simulink library "thc"  (R2021b)
settings: Solver=VariableStepAuto  StartTime=0.0  StopTime=10.0  RelTol=1e-3
undefined symbols (not defined in the file or in its folder): ATHC_APTCQA_X_C, ATHC_APTCQB_X_C, ATHC_dAy_X_C, ATHC_Qeq_X_kmh, ATHC_VbaseC_X_C, ATHC_VbaseC_Y_W, ATHC_VbaseD_X_C, ATHC_VbaseH_X_C, FALSE, KTHC_ACMaxMinT_sec, KTHC_aDeice_K, KTHC_AGSDefLv_K, KTHC_AGSLv1_K, KTHC_AGSLv2_K, KTHC_AGSLv3_K, KTHC_AGSLv4_K, KTHC_AGSLv5_K, KTHC_AirIntUpdateT_sec, KTHC_APTCOneZoneMax_W, KTHC_APTCPeriod_cnt, KTHC_APTCPWMEN_flg, KTHC_APTCQMaxC_W, KTHC_APTCQminC_W, KTHC_APTCQminD_W, KTHC_APTCQminRe1_W, KTHC_APTCQminRe_W, KTHC_APTCQoffT_cnt, KTHC_APTCQonT_cnt, KTHC_APTCRiLeMaxDff_W, KTHC_APTCRiLeMinDff_W, KTHC_BatInTempDef_C, KTHC_bDeice_K, KTHC_CompMaxDeice_rpm, KTHC_CompMinDeice_rpm, KTHC_CompSotxvOp_K, KTHC_CompSotxvOpLow_rpm, KTHC_CompSpdmax_rpm, KTHC_CompSpdmaxBC1_rpm, KTHC_CompSpdmaxBC_rpm, KTHC_CompSpdmid1_rpm, KTHC_CompSpdmid2_rpm, KTHC_CompSpdmid3_rpm, KTHC_CompSpdmid_rpm, KTHC_CompSpdmin_rpm, KTHC_DAPTCQ1_W, KTHC_DAPTCQ2_W, KTHC_DAPTCQ3_W, KTHC_DcChSetTemp_C, KTHC_DehumidityEN_flg, KTHC_DeiceCycTime_K, KTHC_DriveLevelWPTCBAH1_W, KTHC_DriveLevelWPTCBAH2_W, KTHC_DriveLevelWPTCBAH3_W, KTHC_DriveLevelWPTCBAH4_W, KTHC_DriveT1MinBAH_C, KTHC_DriveT2MaxBAH_C, KTHC_DriveT2MinBAH_C, KTHC_DriveT3MaxBAH_C, KTHC_DriveT3MinBAH_C, KTHC_DriveT4MaxBAH_C ... (+372)
libraries: simulink x140
(part 8 of 10)

== stateflow chart thc/THC/ThermalControl/THCM_Conctrl/BlowerCtrl/Enabled Subsystem1/Chart2 ==
  state Voffset [parallel]
    settings: executionOrder=2
    state ACOFF
      state POWERon
        en:Voffset=Vmanual;
        du:Voffset=Vmanual;
      state OFF
        en:Voffset=0;
      (default) -> (junction 8)
      (junction 8) -> POWERon [order 2]
      (junction 8) -> OFF [order 1] : [CabinMode==0||....
          | PwrSta<=3]
      OFF -> POWERon : [CabinMode~=0&&PwrSta>3]
      POWERon -> OFF : [CabinMode==0||....
          | PwrSta<=3]
    state ACON
      state Defrst
        state Manual
          en:Voffset=Vmanual;
          du:Voffset=Vmanual;
        state Auto
          en:Voffset=KTHC_VBlowerdfog_K;
        (default) -> (junction 56)
        (junction 56) -> Voffset.ACON.Defrst.Auto [order 1] : [ACAuto]
        (junction 56) -> Voffset.ACON.Defrst.Manual [order 2]
        Voffset.ACON.Defrst.Manual -> Voffset.ACON.Defrst.Auto : [ACAuto]
        Voffset.ACON.Defrst.Auto -> Voffset.ACON.Defrst.Manual : [!ACAuto]
      state DefrstOFF
        state Auto
          state DontCorrect3
            en:Voffset=KTHC_VBlowerSetLow_K;
          state Vbase1
            en:Voffset=KTHC_VBlowerDcCh_K;
          state Vbase
            en:Voffset=Vbase;
            du:Voffset=Vbase;
          (default) -> (junction 105)
          (junction 105) -> DontCorrect3 [order 1] : [CabinMode==3&&....
              | (ACSubMode==6||ACSubMode==7||ACSubMode==0)]
          Voffset.ACON.DefrstOFF.Auto -> (junction 105) [order 1] : [hasChanged(CabinMode)||....
              | hasChanged(ACSubMode)]
          (junction 105) -> (junction 304) [order 2]
          (junction 304) -> Vbase1 [order 1] : [CabinMode==11]
          (junction 304) -> (junction 293) [order 2]
          (junction 293) -> Voffset.ACON.DefrstOFF.Auto.Vbase
        state Manual
          state DontCorrect
            en:Voffset=Vmanual;
            du:Voffset=Vmanual;
          state Vbase
            en:Voffset=Vbase;
            du:Voffset=Vbase;
          (default) -> (junction 83)
          Voffset.ACON.DefrstOFF.Manual -> (junction 83) [order 1] : [hasChanged(CabinMode)||....
              | hasChanged(ACSubMode)]
          (junction 83) -> DontCorrect [order 1] : [(CabinMode==3&&ACSubMode>=4)||CabinMode==7]
          (junction 83) -> (junction 91) [order 2]
          (junction 91) -> Voffset.ACON.DefrstOFF.Manual.Vbase
        (default) -> (junction 76)
        (junction 76) -> Voffset.ACON.DefrstOFF.Manual [order 2]
        (junction 76) -> Voffset.ACON.DefrstOFF.Auto [order 1] : [ACAuto]
        Voffset.ACON.DefrstOFF.Manual -> Voffset.ACON.DefrstOFF.Auto [order 1] : [ACAuto]
        Voffset.ACON.DefrstOFF.Auto -> Voffset.ACON.DefrstOFF.Manual [order 1] : [!ACAuto]
      (default) -> (junction 58)
      (junction 58) -> Defrst [order 1] : [DfrstReq]
      (junction 58) -> DefrstOFF [order 2]
      DefrstOFF -> Defrst : [DfrstReq]
      Defrst -> DefrstOFF : [!DfrstReq]
    (default) -> ACOFF
    ACOFF -> ACON : [CabinMode>2&&....
        | (CabinMode!=10||....
        | ACSubMode!=1)]
    ACON -> ACOFF : [CabinMode<=2||....
        | (CabinMode==10&&....
        | ACSubMode==1)]
  state VBase [parallel]
    settings: executionOrder=1
    state Cooling
      en:Vbase=VbaseC;
      du:Vbase=VbaseC;
    state Dehumidity
      en:Vbase=VbaseD;
      du:Vbase=VbaseD;
    state Heating
      en:Vbase=VbaseH;
      du:Vbase=VbaseH;
    state Vmanual
      en:Vbase=Vmanual;
      du:Vbase=Vmanual;
    (default) -> (junction 250)
    (junction 254) -> Cooling [order 1] : [CabinMode==3||....
        | (CabinMode==6&&ACSubMode==2)]
    VBase -> (junction 250) : [hasChanged(CabinMode)||....
        | hasChanged(ACAuto)]
    (junction 250) -> (junction 254) [order 1] : [ACAuto]
    (junction 250) -> Vmanual [order 2]
    (junction 254) -> (junction 258) [order 2]
    (junction 258) -> Dehumidity [order 1] : [CabinMode>3&&CabinMode<8]
    (junction 258) -> (junction 263) [order 2]
    (junction 263) -> Heating [order 1] : [CabinMode>=8]
    (junction 263) -> Vmanual [order 2]
  data: ACAuto input; ACSubMode input; CabinMode input; DfrstReq input; VbaseC input; VbaseD input; VbaseH input; Vmanual input; Vbase local double; Voffset output; PwrSta input; KTHC_VBlowerdfog_K input; KTHC_VBlowerMin_K input; KTHC_VBlowerMid_K input; KTHC_VBlowerDcCh_K input; KTHC_VBlowerSetLow_K input

== stateflow chart thc/THC/ThermalControl/THCM_Conctrl/CompCtrl/Enabled Subsystem/Chart ==
  state LV1
    en:DTymin=KTHC_DTymin1_K;
  state LV2
    en:DTymin=KTHC_DTymin2_K;
  state LV3
    en:DTymin=KTHC_DTymin3_K;
  state LV4
    en:DTymin=KTHC_DTymin4_K;
  state LV5
    en:DTymin=KTHC_DTymin5_K;
  (default) -> (junction 8)
  (junction 8) -> LV1 [order 1] : [Tamb<KTHC_T1Maxamb_C]
  (junction 8) -> (junction 9) [order 2]
  LV1 -> LV2 : [Tamb>KTHC_T1Maxamb_C]
  LV2 -> LV1 [order 2] : [Tamb<KTHC_T2Minamb_C]
  (junction 9) -> LV2 [order 1] : [Tamb<KTHC_T2Maxamb_C]
  (junction 9) -> (junction 10) [order 2]
  LV2 -> LV3 [order 1] : [Tamb>KTHC_T2Maxamb_C]
  LV3 -> LV2 [order 2] : [Tamb<KTHC_T3Minamb_C]
  (junction 10) -> LV3 [order 1] : [Tamb<KTHC_T3Maxamb_C]
  (junction 10) -> (junction 11) [order 2]
  LV3 -> LV4 [order 1] : [Tamb>KTHC_T3Maxamb_C]
  LV4 -> LV3 [order 2] : [Tamb<KTHC_T4Minamb_C]
  (junction 11) -> LV4 [order 1] : [Tamb<KTHC_T4Maxamb_C]
  (junction 11) -> (junction 12) [order 2]
  LV4 -> LV5 [order 1] : [Tamb>KTHC_T4Maxamb_C]
  LV5 -> LV4 : [Tamb<KTHC_T5Minamb_C]
  (junction 12) -> LV5
  data: Tamb input; KTHC_DTymin1_K input; KTHC_DTymin2_K input; KTHC_DTymin3_K input; KTHC_DTymin4_K input; KTHC_DTymin5_K input; KTHC_T1Maxamb_C input; KTHC_T2Maxamb_C input; KTHC_T3Maxamb_C input; KTHC_T4Maxamb_C input; KTHC_T2Minamb_C input; KTHC_T3Minamb_C input; KTHC_T4Minamb_C input; KTHC_T5Minamb_C input; DTymin output double

== stateflow chart thc/THC/ThermalControl/THCM_Conctrl/APTC/Chart ==
  state APTCPro_FrLe [parallel]
    settings: executionOrder=1
    state Derating
      state State2
        (default) -> (junction 23)
        APTCPro_FrLe.Derating.State2 -> (junction 23) [order 1]
        (junction 23) -> (junction 26) [order 1] : [FD_FrLeAPTCHeatPwr_Cmd>KTHC_DAPTCQ1_W]{FD_FrLeAPTCHeatPwr_Cmd=FD_FrLeAPTCHeatPwr_Cmd-KTHC_DAPTCQ1_W;}
        (junction 23) -> (junction 28) [order 2] : {FD_FrLeAPTCHeatPwr_Cmd=0;}
      state State3
        (default) -> (junction 31)
        APTCPro_FrLe.Derating.State3 -> (junction 31) [order 1]
        (junction 31) -> (junction 32) [order 1] : [FD_FrLeAPTCHeatPwr_Cmd>KTHC_DAPTCQ2_W]{FD_FrLeAPTCHeatPwr_Cmd=FD_FrLeAPTCHeatPwr_Cmd-KTHC_DAPTCQ2_W;}
        (junction 31) -> (junction 33) [order 2] : {FD_FrLeAPTCHeatPwr_Cmd=0;}
      state State4
        (default) -> (junction 39)
        APTCPro_FrLe.Derating.State4 -> (junction 39) [order 1]
        (junction 39) -> (junction 40) [order 1] : [FD_FrLeAPTCHeatPwr_Cmd>KTHC_DAPTCQ3_W]{FD_FrLeAPTCHeatPwr_Cmd=FD_FrLeAPTCHeatPwr_Cmd-KTHC_DAPTCQ3_W;}
        (junction 39) -> (junction 41) [order 2] : {FD_FrLeAPTCHeatPwr_Cmd=0;}
      state State5
      (default) -> APTCPro_FrLe.Derating.State2
      APTCPro_FrLe.Derating.State3 -> APTCPro_FrLe.Derating.State2 [order 1] : [Tventmax_FrLe>KTHC_TventL1_C]
      APTCPro_FrLe.Derating.State2 -> APTCPro_FrLe.Derating.State3 [order 1] : [Tventmax_FrLe<KTHC_TventL2_C]
      APTCPro_FrLe.Derating.State4 -> APTCPro_FrLe.Derating.State3 [order 1] : [Tventmax_FrLe>KTHC_TventL2_C]
      APTCPro_FrLe.Derating.State3 -> APTCPro_FrLe.Derating.State4 [order 2] : [Tventmax_FrLe<KTHC_TventL3_C]
      APTCPro_FrLe.Derating.State5 -> APTCPro_FrLe.Derating.State4 : [Tventmax_FrLe>KTHC_TventL3_C]
      APTCPro_FrLe.Derating.State4 -> APTCPro_FrLe.Derating.State5 [order 2] : [Tventmax_FrLe<KTHC_TventL4_C]
    state PICtrl
      en:FD_FrLeAPTCHeatPwr_Cmd=FD_FrLeAPTC_Cmd;
      du:FD_FrLeAPTCHeatPwr_Cmd=FD_FrLeAPTC_Cmd;
      state Normal
        en:CtrlReset=0;
      state ResetController
        en:CtrlReset=1;
      (default) -> APTCPro_FrLe.PICtrl.Normal
      APTCPro_FrLe.PICtrl.ResetController -> APTCPro_FrLe.PICtrl.Normal
    (default) -> APTCPro_FrLe.PICtrl
    APTCPro_FrLe.PICtrl -> APTCPro_FrLe.Derating : [Tventmax_FrLe>KTHC_TventL1_C]
    APTCPro_FrLe.Derating -> APTCPro_FrLe.PICtrl [order 2] : [FD_FrLeAPTCHeatPwr_Cmd>FD_FrLeAPTC_Cmd]
    APTCPro_FrLe.Derating -> APTCPro_FrLe.PICtrl.ResetController [order 1] : [Tventmax_FrLe<KTHC_TventL5_C]
  state APTCPro_FrRi [parallel]
    settings: executionOrder=2
    state Derating
      state State2
        (default) -> (junction 87)
        APTCPro_FrRi.Derating.State2 -> (junction 87) [order 1]
        (junction 87) -> (junction 88) [order 1] : [FD_FrRiAPTCHeatPwr_Cmd>KTHC_DAPTCQ1_W]{FD_FrRiAPTCHeatPwr_Cmd=FD_FrRiAPTCHeatPwr_Cmd-KTHC_DAPTCQ1_W;}
        (junction 87) -> (junction 89) [order 2] : {FD_FrRiAPTCHeatPwr_Cmd=0;}
      state State3
        (default) -> (junction 58)
        APTCPro_FrRi.Derating.State3 -> (junction 58) [order 1]
        (junction 58) -> (junction 59) [order 1] : [FD_FrRiAPTCHeatPwr_Cmd>KTHC_DAPTCQ2_W]{FD_FrRiAPTCHeatPwr_Cmd=FD_FrRiAPTCHeatPwr_Cmd-KTHC_DAPTCQ2_W;}
        (junction 58) -> (junction 60) [order 2] : {FD_FrRiAPTCHeatPwr_Cmd=0;}
      state State4
        (default) -> (junction 78)
        APTCPro_FrRi.Derating.State4 -> (junction 78) [order 1]
        (junction 78) -> (junction 79) [order 1] : [FD_FrRiAPTCHeatPwr_Cmd>KTHC_DAPTCQ3_W]{FD_FrRiAPTCHeatPwr_Cmd=FD_FrRiAPTCHeatPwr_Cmd-KTHC_DAPTCQ3_W;}
        (junction 78) -> (junction 80) [order 2] : {FD_FrRiAPTCHeatPwr_Cmd=0;}
      state State5
      (default) -> APTCPro_FrRi.Derating.State2
      APTCPro_FrRi.Derating.State3 -> APTCPro_FrRi.Derating.State2 [order 1] : [Tventmax_FrRi>KTHC_TventL1_C]
      APTCPro_FrRi.Derating.State2 -> APTCPro_FrRi.Derating.State3 [order 1] : [Tventmax_FrRi<KTHC_TventL2_C]
      APTCPro_FrRi.Derating.State4 -> APTCPro_FrRi.Derating.State3 [order 1] : [Tventmax_FrRi>KTHC_TventL2_C]
      APTCPro_FrRi.Derating.State3 -> APTCPro_FrRi.Derating.State4 [order 2] : [Tventmax_FrRi<KTHC_TventL3_C]
      APTCPro_FrRi.Derating.State5 -> APTCPro_FrRi.Derating.State4 : [Tventmax_FrRi>KTHC_TventL3_C]
      APTCPro_FrRi.Derating.State4 -> APTCPro_FrRi.Derating.State5 [order 2] : [Tventmax_FrRi<KTHC_TventL4_C]
    state PICtrl
      en:FD_FrRiAPTCHeatPwr_Cmd=FD_FrRiAPTC_Cmd;
      du:FD_FrRiAPTCHeatPwr_Cmd=FD_FrRiAPTC_Cmd;
      state Normal
        en:CtrlReset=0;
      state ResetController
        en:CtrlReset=1;
      (default) -> APTCPro_FrRi.PICtrl.Normal
      APTCPro_FrRi.PICtrl.ResetController -> APTCPro_FrRi.PICtrl.Normal
    (default) -> APTCPro_FrRi.PICtrl
    APTCPro_FrRi.PICtrl -> APTCPro_FrRi.Derating : [Tventmax_FrRi>KTHC_TventL1_C]
    APTCPro_FrRi.Derating -> APTCPro_FrRi.PICtrl [order 2] : [FD_FrRiAPTCHeatPwr_Cmd>FD_FrRiAPTC_Cmd]
    APTCPro_FrRi.Derating -> APTCPro_FrRi.PICtrl.ResetController [order 1] : [Tventmax_FrRi<KTHC_TventL5_C]
  state APTCPro_Rr [parallel]
    settings: executionOrder=3
    state Derating
      state State2
        (default) -> (junction 125)
        APTCPro_Rr.Derating.State2 -> (junction 125) [order 1]
        (junction 125) -> (junction 126) [order 1] : [FD_RrAPTCHeatPwr_Cmd>KTHC_DAPTCQ1_W]{FD_RrAPTCHeatPwr_Cmd=FD_RrAPTCHeatPwr_Cmd-KTHC_DAPTCQ1_W;}
        (junction 125) -> (junction 127) [order 2] : {FD_RrAPTCHeatPwr_Cmd=0;}
      state State3
        (default) -> (junction 96)
        APTCPro_Rr.Derating.State3 -> (junction 96) [order 1]
        (junction 96) -> (junction 97) [order 1] : [FD_RrAPTCHeatPwr_Cmd>KTHC_DAPTCQ2_W]{FD_RrAPTCHeatPwr_Cmd=FD_RrAPTCHeatPwr_Cmd-KTHC_DAPTCQ2_W;}
        (junction 96) -> (junction 98) [order 2] : {FD_RrAPTCHeatPwr_Cmd=0;}
      state State4
        (default) -> (junction 116)
        APTCPro_Rr.Derating.State4 -> (junction 116) [order 1]
        (junction 116) -> (junction 117) [order 1] : [FD_RrAPTCHeatPwr_Cmd>KTHC_DAPTCQ3_W]{FD_RrAPTCHeatPwr_Cmd=FD_RrAPTCHeatPwr_Cmd-KTHC_DAPTCQ3_W;}
        (junction 116) -> (junction 118) [order 2] : {FD_RrAPTCHeatPwr_Cmd=0;}
      state State5
      (default) -> APTCPro_Rr.Derating.State2
      APTCPro_Rr.Derating.State3 -> APTCPro_Rr.Derating.State2 [order 1] : [Tventmax_Rr>KTHC_TventL1_C]
      APTCPro_Rr.Derating.State2 -> APTCPro_Rr.Derating.State3 [order 1] : [Tventmax_Rr<KTHC_TventL2_C]
      APTCPro_Rr.Derating.State4 -> APTCPro_Rr.Derating.State3 [order 1] : [Tventmax_Rr>KTHC_TventL2_C]
      APTCPro_Rr.Derating.State3 -> APTCPro_Rr.Derating.State4 [order 2] : [Tventmax_Rr<KTHC_TventL3_C]
      APTCPro_Rr.Derating.State5 -> APTCPro_Rr.Derating.State4 : [Tventmax_Rr>KTHC_TventL3_C]
      APTCPro_Rr.Derating.State4 -> APTCPro_Rr.Derating.State5 [order 2] : [Tventmax_Rr<KTHC_TventL4_C]
    state PICtrl
      en:FD_RrAPTCHeatPwr_Cmd=FD_RrAPTC_Cmd;
      du:FD_RrAPTCHeatPwr_Cmd=FD_RrAPTC_Cmd;
      state Normal
        en:CtrlReset=0;
      state ResetController
        en:CtrlReset=1;
      (default) -> APTCPro_Rr.PICtrl.Normal
      APTCPro_Rr.PICtrl.ResetController -> APTCPro_Rr.PICtrl.Normal
    (default) -> APTCPro_Rr.PICtrl
    APTCPro_Rr.PICtrl -> APTCPro_Rr.Derating : [Tventmax_Rr>KTHC_TventL1_C]
    APTCPro_Rr.Derating -> APTCPro_Rr.PICtrl [order 2] : [FD_RrAPTCHeatPwr_Cmd>FD_RrAPTC_Cmd]
    APTCPro_Rr.Derating -> APTCPro_Rr.PICtrl.ResetController [order 1] : [Tventmax_Rr<KTHC_TventL5_C]
  data: FD_FrLeAPTC_Cmd input; FD_FrRiAPTC_Cmd input; FD_RrAPTC_Cmd input; Tventmax_FrLe input; Tventmax_FrRi input; Tventmax_Rr input; KTHC_TventL1_C input; KTHC_TventL2_C input; KTHC_TventL3_C input; KTHC_TventL4_C input; KTHC_TventL5_C input; KTHC_DAPTCQ1_W input; KTHC_DAPTCQ2_W input; KTHC_DAPTCQ3_W input; FD_FrLeAPTCHeatPwr_Cmd output double; FD_FrRiAPTCHeatPwr_Cmd output double; FD_RrAPTCHeatPwr_Cmd output double; CtrlReset output boolean

== stateflow chart thc/THC/ThermalControl/THCM_Conctrl/Chart1 ==
  state TambLevel
    state WaitForUpdate
    (default) -> (junction 43)
    WaitForUpdate -> (junction 43) [order 4] : [hasChanged(ECOSW)]
    (junction 43) -> (junction 19)
    WaitForUpdate -> (junction 19) [order 1] : [hasChanged(SetTempZon1St_CMD)]
    (junction 19) -> (junction 25)
    WaitForUpdate -> (junction 25) [order 2] : [hasChanged(SetTempZon2St_CMD)]
    (junction 25) -> (junction 21)
    WaitForUpdate -> (junction 21) [order 3] : [after(KTHC_ECOTambLVT_sec*10,tick)]
    (junction 21) -> (junction 46)
    (junction 46) -> WaitForUpdate [order 1] : [!ECOSW]{alpha=0;beta=0;sigSetTempZon1Stadj=sigSetTempZon1St;sigSetTempZon2Stadj=sigSetTempZon2St;}
    (junction 46) -> (junction 5) [order 2]
    (junction 5) -> (junction 29) [order 1] : [Tamb<KTHC_ECOTambLV1_C]{alpha=KTHC_ECOalpha1_K;beta=KTHC_ECObeta1_K;}
    (junction 5) -> (junction 7) [order 2]
    (junction 29) -> (junction 31)
    (junction 7) -> (junction 31) [order 1] : [Tamb<KTHC_ECOTambLV2_C]{alpha=KTHC_ECOalpha2_K;beta=KTHC_ECObeta2_K;}
    (junction 7) -> (junction 10) [order 2]
    (junction 31) -> (junction 34)
    (junction 10) -> (junction 34) [order 1] : [Tamb<KTHC_ECOTambLV3_C]{alpha=KTHC_ECOalpha3_K;beta=KTHC_ECObeta3_K;}
    (junction 10) -> (junction 13) [order 2]
    (junction 34) -> (junction 37)
    (junction 13) -> (junction 37) [order 1] : [Tamb<KTHC_ECOTambLV4_C]{alpha=KTHC_ECOalpha4_K;beta=KTHC_ECObeta4_K;}
    (junction 13) -> (junction 16) [order 2]
    (junction 37) -> (junction 40)
    (junction 16) -> (junction 40) [order 1] : [Tamb<KTHC_ECOTambLV5_C]{alpha=KTHC_ECOalpha5_K;beta=KTHC_ECObeta5_K;}
    (junction 16) -> (junction 110) [order 2]
    (junction 40) -> (junction 97)
    (junction 110) -> (junction 97) [order 1] : [Tamb<KTHC_ECOTambLV6_C]{alpha=KTHC_ECOalpha6_K;beta=KTHC_ECObeta6_K;}
    (junction 110) -> (junction 107) [order 2]
    (junction 97) -> (junction 95)
    (junction 107) -> (junction 95) [order 1] : [Tamb<KTHC_ECOTambLV7_C]{alpha=KTHC_ECOalpha7_K;beta=KTHC_ECObeta7_K;}
    (junction 107) -> (junction 103) [order 2]
    (junction 95) -> (junction 100)
    (junction 103) -> (junction 100) [order 1] : [Tamb<KTHC_ECOTambLV8_C]{alpha=KTHC_ECOalpha8_K;beta=KTHC_ECObeta8_K;}
    (junction 103) -> (junction 94) [order 2]
    (junction 100) -> (junction 102)
    (junction 94) -> (junction 102) : {alpha=KTHC_ECOalpha9_K;beta=KTHC_ECObeta9_K;}
    (junction 102) -> (junction 54) [order 1] : [sigSetTempZon1St<Tamb]
        | {sigSetTempZon1Stadj=sigSetTempZon1St-(sigSetTempZon1St-Tamb)*alpha;}
    (junction 102) -> (junction 55) [order 2]
    (junction 54) -> (junction 57)
    (junction 55) -> (junction 57) : {sigSetTempZon1Stadj=sigSetTempZon1St-(sigSetTempZon1St-Tamb)*beta;}
    (junction 57) -> WaitForUpdate [order 1] : [sigSetTempZon2St<Tamb]
        | {sigSetTempZon2Stadj=sigSetTempZon2St-(sigSetTempZon2St-Tamb)*alpha;}
    (junction 57) -> (junction 62) [order 2]
    (junction 62) -> WaitForUpdate : {sigSetTempZon2Stadj=sigSetTempZon2St-(sigSetTempZon2St-Tamb)*beta;}
  data: KTHC_ECOTambLV1_C input; KTHC_ECOTambLV2_C input; KTHC_ECOTambLV3_C input; KTHC_ECOTambLV4_C input; KTHC_ECOTambLV5_C input; KTHC_ECOTambLV6_C input; KTHC_ECOTambLV7_C input; KTHC_ECOTambLV8_C input; KTHC_ECOTambLVT_sec input; KTHC_ECOalpha1_K input; KTHC_ECOalpha2_K input; KTHC_ECOalpha3_K input; KTHC_ECOalpha4_K input; KTHC_ECOalpha5_K input; KTHC_ECOalpha6_K input; KTHC_ECOalpha7_K input; KTHC_ECOalpha8_K input; KTHC_ECObeta1_K input; KTHC_ECObeta2_K input; KTHC_ECObeta3_K input; KTHC_ECObeta4_K input; KTHC_ECObeta5_K input; KTHC_ECOalpha9_K input; KTHC_ECObeta6_K input; KTHC_ECObeta7_K input; KTHC_ECObeta8_K input; KTHC_ECObeta9_K input; Tamb input; sigSetTempZon1St input; SetTempZon1St_CMD input; sigSetTempZon1Stadj output double; alpha local double; beta local double; sigSetTempZon2St input; SetTempZon2St_CMD input; sigSetTempZon2Stadj output double; ECOSW input

== stateflow chart thc/THC/ThermalControl/THCM_Conctrl/CompCtrl/Enabled Subsystem1/Chart ==
  state Level1
    en:Bat_In_TempSetPoint=KTHC_T1winSetpointBC_C;
  state Level2
    en:Bat_In_TempSetPoint=KTHC_T2winSetpointBC_C;
  state Level3
    en:Bat_In_TempSetPoint=KTHC_T3winSetpointBC_C;
  state Level4
    en:Bat_In_TempSetPoint=KTHC_T4winSetpointBC_C;
  state Level5
    en:Bat_In_TempSetPoint=KTHC_T5winSetpointBC_C;
  (default) -> Level1
  Level1 -> Level2 : [TBMax>KTHC_T1MaxBC_C]
  Level2 -> Level1 [order 2] : [TBMax<KTHC_T2MinBC_C]
  Level2 -> Level3 [order 1] : [TBMax>KTHC_T2MaxBC_C]
  Level3 -> Level2 [order 2] : [TBMax<KTHC_T3MinBC_C]
  Level3 -> Level4 [order 1] : [TBMax>KTHC_T3MaxBC_C]
  Level4 -> Level3 [order 1] : [TBMax<KTHC_T4MinBC_C]
  Level4 -> Level5 [order 2] : [TBMax>KTHC_T4MaxBC_C]
  Level5 -> Level4 : [TBMax<KTHC_T5MinBC_C]
  data: TBMax input; Bat_In_TempSetPoint output; KTHC_T1MaxBC_C input; KTHC_T2MinBC_C input; KTHC_T2MaxBC_C input; KTHC_T3MinBC_C input; KTHC_T3MaxBC_C input; KTHC_T4MinBC_C input; KTHC_T4MaxBC_C input; KTHC_T5MinBC_C input; KTHC_T1winSetpointBC_C input; KTHC_T2winSetpointBC_C input; KTHC_T3winSetpointBC_C input; KTHC_T4winSetpointBC_C input; KTHC_T5winSetpointBC_C input

== stateflow chart thc/THC/ThermalControl/THCM_Conctrl/APTC/Chart1 ==
  state OFF
    en:APTCset=0;
  state ONOFF
    state ON
      en:APTCset=KTHC_APTCQminC_W;
    state OFF
      en:APTCset=0;
    (default) -> ON
    ON -> ONOFF.OFF : [after(KTHC_APTCQonT_cnt,tick)]
    ONOFF.OFF -> ON : [after(KTHC_APTCQoffT_cnt,tick)]
  (default) -> OFF
  OFF -> ONOFF : [APTCPID==8]
  ONOFF -> OFF : [APTCPID!=8]
  data: KTHC_APTCQminC_W input; APTCPID input; KTHC_APTCQonT_cnt input; KTHC_APTCQoffT_cnt input; APTCset output double
